simulink model "HQ1"  (R2018a)
settings: Solver=ode45  StartTime=0.0  StopTime=10.0  MaxStep=0.1  MinStep=0.1  RelTol=1e-3
InitFcn:
  | var_HQ
values from neighbouring files (symbols this model uses):
  lev_max = 1000    [var_HQ.m]
  rou = 0.9    [var_HQ.m]
  u_min = 0.05    [var_HQ.m]
settings Model: Creator=Administrator  LastModifiedBy=Administrator

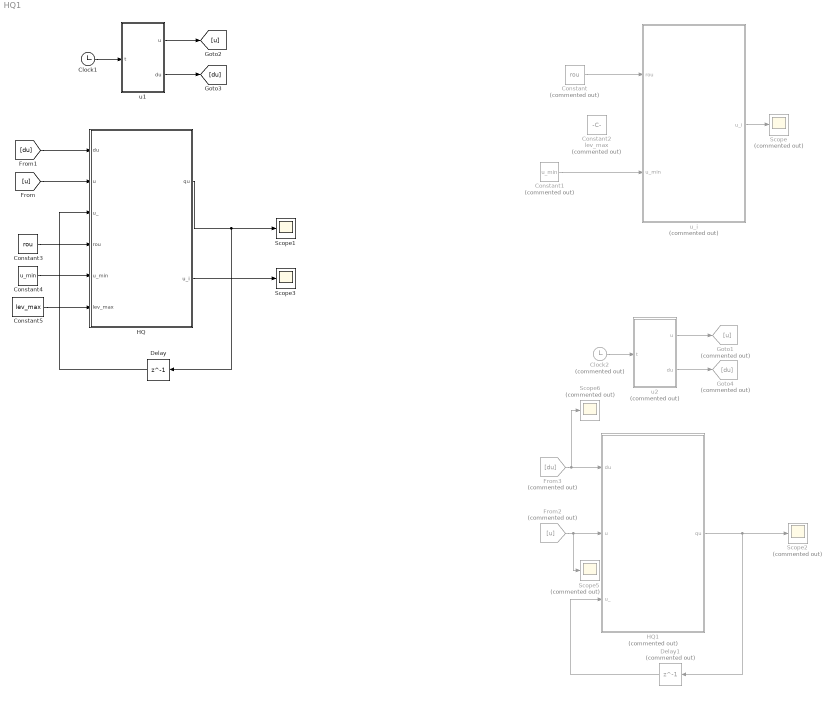
== system HQ1 ==
  Clock1 : Clock
  Clock2 : Clock  Commented=on
  Constant : Constant  Commented=on  Value=rou
  Constant1 : Constant  Commented=on  Value=u_min
  Constant2 : Constant  Commented=on  Value=lev_max
  Constant3 : Constant  Value=rou
  Constant4 : Constant  Value=u_min
  Constant5 : Constant  Value=lev_max
  Delay : Delay  DelayLength=1  InitialCondition=0
  Delay1 : Delay  Commented=on  DelayLength=1  InitialCondition=0
  From2 : From  Commented=on  GotoTag=u
  From3 : From  Commented=on  GotoTag=du
  Goto1 : Goto  Commented=on  GotoTag=u
  Goto4 : Goto  Commented=on  GotoTag=du
  HQ : MATLAB Function  TreatAsAtomicUnit=on
  HQ1 : MATLAB Function  Commented=on  TreatAsAtomicUnit=on
  Scope{,2,5..6} (4 alike) : Scope  Commented=on
  Scope1 : Scope
  Scope3 : Scope
  u1 : MATLAB Function  TreatAsAtomicUnit=on
  u2 : MATLAB Function  Commented=on  TreatAsAtomicUnit=on
  u_i : MATLAB Function  Commented=on  TreatAsAtomicUnit=on
  wires:
  Constant/1 -> u_i/1(rou)
  Constant1/1 -> u_i/2(u_min)
  u_i/1(u_i) -> Scope/1
  HQ/1(qu) -> Delay/1, Scope1/1
  u1/2(du) -> [du]
  u1/1(u) -> [u]
  Clock1/1 -> u1/1(t)
  Delay/1 -> HQ/3(u_)
  [u] -> HQ/2(u)
  [du] -> HQ/1(du)
  Clock2/1 -> u2/1(t)
  u2/2(du) -> Goto4/1
  u2/1(u) -> Goto1/1
  HQ1/1(qu) -> Delay1/1, Scope2/1
  Delay1/1 -> HQ1/3(u_)
  From3/1 -> Scope6/1, HQ1/1(du)
  From2/1 -> Scope5/1, HQ1/2(u)
  Constant5/1 -> HQ/6(lev_max)
  Constant4/1 -> HQ/5(u_min)
  Constant3/1 -> HQ/4(rou)
  HQ/2(u_i) -> Scope3/1

== matlab function HQ1/u_i ==
  data: u_i output; rou input; u_min input
function u_i = fcn(rou,u_min)

lev_max=1000;
u_i=zeros(length(1:lev_max),1);
ii=1:lev_max;
u_i(ii,1)=rou.^(1-ii).*u_min;

== matlab function HQ1/HQ ==
  data: du input; qu output; u input; u_ input; rou input; u_min input; lev_max input; u_i output
function [qu,u_i] = fcn(du,u,u_,rou,u_min,lev_max)


% rou=(1-delta)/(1+delta);
% i=0;
% lev=1:lev_max;
% while abs(u)>=rou^(1-i-1)
%         i=i+1;
% end
delta=(1-rou)/(1+rou);
flag=sign(du);
qu=0;
u_i=-1;
for i=1:lev_max
    u_i=(rou^(1-i))*u_min;
    switch flag
    case -1
        if (abs(u) > (u_i/(1+delta)))&&(abs(u) <= u_i)
            qu=u_i*sign(u);
            break;
        elseif (abs(u) > u_i)&&(abs(u) <= u_i/(1-delta))
            qu=u_i*(1+delta)*sign(u);
            break;
        elseif (abs(u) >= 0)&&(abs(u) < u_min/(1+delta))
            qu=0;
            break;
        end
    case 1
        if (abs(u)>=u_min)&&(abs(u) > u_i)&&(abs(u) <= u_i/(1-delta))
            qu=u_i*sign(u);
            break;
        elseif (abs(u)>=u_min)&&(abs(u) > u_i/(1-delta))&&(abs(u) <= u_i*(1+delta)/(1-delta))
            qu=u_i*(1+delta)*sign(u);
            break;
%         elseif (abs(u) >= u_min/(1+delta))&&(abs(u) <= u_min)
%             qu=0;
%             break;
        elseif (abs(u) >= 0)&&(abs(u) <= u_min)
            qu=0;
            break;
        end
    case 0
        qu=u_;
        break;
    end
end

== matlab function HQ1/HQ1 ==
  data: du input; qu output; u input; u_ input
function qu = fcn(du,u,u_)

delta=0.2;

umin=0.02;
rho=(1-delta)/(1+delta);
i=0;
while abs(u)>=((rho^(1-i-1))*umin)
        i=i+1;
end
uj=(rho^(1-i))*umin;
if du>0
     if (umin<=abs(u))&&(uj<abs(u))&&(abs(u)<=uj/(1-delta))
         qu=uj*sign(u);
     elseif (umin<=abs(u))&&(uj/(1-delta)<abs(u))&&(abs(u)<=uj*(1+delta)/(1-delta))
              qu=uj*(1+delta)*sign(u);
%      elseif (0<=abs(u))&&(abs(u)<=umin)
%                  qu=0;
     elseif (abs(u) >= umin/(1+delta))&&(abs(u) <= umin)
                 qu=0;
     else
         qu=0;
     end
elseif du<0
     if (uj/(1-delta)<abs(u))&&(abs(u)<=(uj*(1+delta))/(1-delta))
         qu=rho^(1-(i+1))*umin*sign(u);
     elseif (umin<=abs(u))&&(uj<abs(u))&&(abs(u)<=uj/(1-delta))
             qu=uj*(1+delta)*sign(u); 
     elseif (0<=abs(u))&&(abs(u)<(umin/(1+delta)))
                 qu=0;
     else
         qu=0;
     end

elseif du==0
     qu=u_;
else
    qu=0;
 end

== matlab function HQ1/u1 ==
  data: t input; u output; du output
function [u,du] = fcn(t)

u=sin(t);
du=cos(t);

== matlab function HQ1/u2 ==
  data: t input; u output; du output
function [u,du] = fcn(t)

u=cos(t);
du=sin(t);
